simulink model "Ass_5_ex"  (R2022a)
settings: Solver=FixedStepAuto  StartTime=0.0  StopTime=inf  FixedStep=0.2  RelTol=1e-3
settings Model: Creator=ArriGE66  LastModifiedBy=ArriGE66

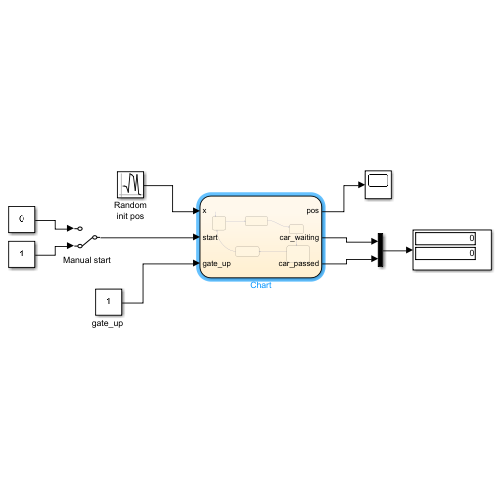
[thumbnail: Simulink's stored preview of the top-level diagram]
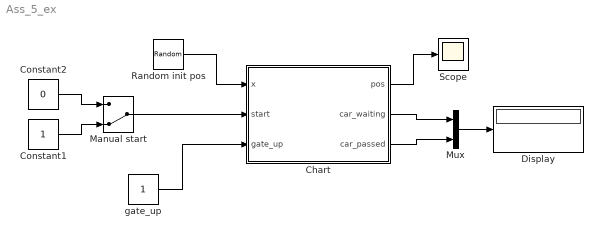
== system Ass_5_ex ==
  Chart : Stateflow chart  TreatAsAtomicUnit=on
  Constant1 : Constant
  Constant2 : Constant  Value=0
  Display : Display
  Manual start : ManualSwitch  CurrentSetting=0
  Mux : Mux  Inputs=2
  Random init pos : RandomNumber  Mean=-15  Variance=5
  Scope : Scope
  "gate_up " : Constant
  wires:
  Random init pos/1 -> Chart/1(x)
  Constant1/1 -> Manual start/2
  Constant2/1 -> Manual start/1
  Manual start/1 -> Chart/2(start)
  "gate_up "/1 -> Chart/3(gate_up)
  Chart/1(pos) -> Scope/1
  Mux/1 -> Display/1
  Chart/2(car_waiting) -> Mux/1
  Chart/3(car_passed) -> Mux/2

== stateflow chart Ass_5_ex/Chart ==
  state idle
    init=x;
    pos=init;
    car_waiting=0;
    car_passed=0;
  state approaching
    pos=init+v*elapsed(sec);
  state stop
    tmp=pos;
    car_waiting=1;
    car_passed=0;
  state pass
    pos=tmp+v*elapsed(sec);
    car_waiting=0;
    ex:
    pos=tmp+v*elapsed(sec);
    tmp=pos;
  state passed
    pos=tmp+v*elapsed(sec);
    car_passed=1;
  (default) -> idle
  approaching -> stop : [pos>=0]
  idle -> approaching : [start==1]
  passed -> idle : [after(10,sec)]
  stop -> pass : [gate_up==1]
  pass -> passed : [pos>= gate_end]
  data: gate_end local =3; v local double =1; pos output; car_waiting output; car_passed output; init local; x input; start input; gate_up input; tmp local
